simulink model "simulation_PID"  (R2020a)
settings: Solver=VariableStepAuto  StartTime=0.0  StopTime=100  RelTol=1e-3
libraries: simulink x1
settings Model: Creator=Ayush Agrawal  LastModifiedBy=Ayush Agrawal

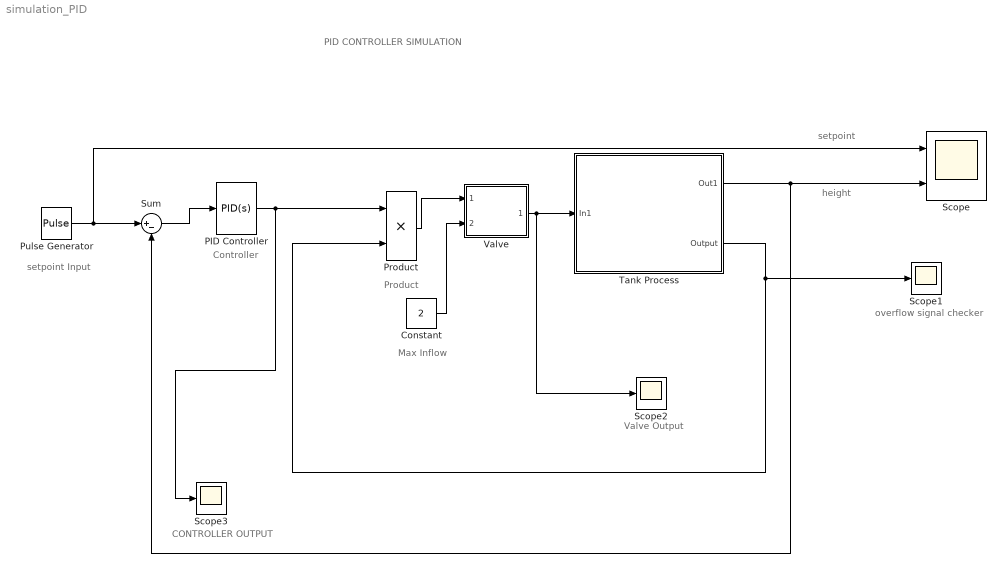
== system simulation_PID ==
  note: PID CONTROLLER SIMULATION
  note: CONTROLLER OUTPUT
  note: Product
  note: Controller
  note: Valve Output
  note: setpoint Input
  note: Max Inflow
  note: height
  note: setpoint
  note: overflow signal checker
  Constant : Constant  Value=2
  PID Controller : simulink/Continuous/PID Controller  Controller=PID  Form=Parallel  TimeDomain=Continuous-time  UseExternalTs=off  SampleTime=-1  IntegratorMethod=Forward Euler  FilterMethod=Forward Euler  ControllerParametersSource=internal  P=160  I=-2.93  D=16  UseFilter=on  N=100  TunerSelectOption=Transfer Function Based (PID Tuner App)  InitialConditionSource=internal  InitialConditionForIntegrator=0  InitialConditionForFilter=0  DifferentiatorICPrevScaledInput=0  ExternalReset=none  TrackingMode=off  Kt=1  LimitOutput=off  UpperSaturationLimit=inf  LowerSaturationLimit=-inf  LinearizeAsGain=on  AntiWindupMode=none  Kb=1  POutMin=[]  POutMax=[]  IOutMin=[]  IOutMax=[]  DOutMin=[]  DOutMax=[]  NOutMin=[]  NOutMax=[]  SumOutMin=[]  SumOutMax=[]  SaturationOutMin=[]  SaturationOutMax=[]  PParamMin=[]  PParamMax=[]  IParamMin=[]  IParamMax=[]  DParamMin=[]  DParamMax=[]  NParamMin=[]  NParamMax=[]  KbParamMin=[]  KbParamMax=[]  KtParamMin=[]  KtParamMax=[]  KbOutMin=[]  KbOutMax=[]  KtOutMin=[]  KtOutMax=[]  IntegratorOutMin=[]  IntegratorOutMax=[]  FilterOutMin=[]  FilterOutMax=[]  SumI1OutMin=[]  SumI1OutMax=[]  SumI2OutMin=[]  SumI2OutMax=[]  SumI3OutMin=[]  SumI3OutMax=[]  SumI4OutMin=[]  SumI4OutMax=[]  SumDOutMin=[]  SumDOutMax=[]  DifferentiatorOutMin=[]  DifferentiatorOutMax=[]  FilterDiffOutCoefMin=[]  FilterDiffOutCoefMax=[]  ReciprocalOutMin=[]  ReciprocalOutMax=[]  SumDenOutMin=[]  SumDenOutMax=[]  SumNumOutMin=[]  SumNumOutMax=[]  DivideOutMin=[]  DivideOutMax=[]  UdiffTsProdOutMin=[]  UdiffTsProdOutMax=[]  NTsProdOutMin=[]  NTsProdOutMax=[]  UintegralTsProdOutMin=[]  UintegralTsProdOutMax=[]  UngainTsProdOutMin=[]  UngainTsProdOutMax=[]  IntegratorContinuousStateAttributes=''  IntegratorStateMustResolveToSignalObject=off  IntegratorRTWStateStorageClass=Auto  FilterContinuousStateAttributes=''  FilterStateMustResolveToSignalObject=off  FilterRTWStateStorageClass=Auto  ParallelPVariant=InternalParameters  IdealPVariant=Disabled  IVariant=InternalParameters  DVariant=InternalParameters  IntegratorVariant=Continuous  SatVariant=Disabled  AWVariant=Passthrough  PCopyVariant=Disabled  TRVariant=Disabled  FdbkBlocksVariant=Forward  IdealPFdbkVariant=Disabled  SatFdbkVariant=Disabled  DerivativeFilterVariant=ContFilter  NVariant=InternalParameters  NCopyVariant=Disabled  FilterICVariant=InternalICsFilter  IntegratorICVariant=InternalICs  ExternalResetVariant=Disabled  TRSumVariant=Passthrough  SumFdbkVariant=Disabled  SumVariant=Sum_PID  TsampFilterVariant=InternalTs  TsampNgainVariant=Passthrough  TsampIntegralVariant=Passthrough
  Product : Product
  Pulse Generator : DiscretePulseGenerator  PulseType=Time based  Period=100  PulseWidth=50
  Scope : Scope  NumInputPorts=2
  Scope1 : Scope
  Scope2 : Scope
  Scope3 : Scope
  Sum : Sum  Inputs=|+-
  Tank Process : Subsystem  mask{ht=10, Tarea=0.4, Oarea=0.04, initialHt=0.0, overflowLimit=0}
      mask prompts: ht "Height of Tank(m)"; Tarea "Tank Area (m^2)"; Oarea "Outflow Cross-Section Area(m^2)"; initialHt "Initial Level Height(m)"; overflowLimit "Overflow Sensor distance from top(m)"
      mask Display: image('C:\Users\Ayush Agrawal\Downloads\94-943202_intermediate-practice-problems-online-brilliant-you-filling-water.png'); % Use "Edit Image" on toolstrip to change.
  Valve : Subsystem  mask(Valve){InitialPosition=0}
      mask prompts: InitialPosition "Initial position [0=closed 1=open]:"
      mask help: Valve
      mask Display: disp('VALVE')
  wires:
  Pulse Generator/1 -> Sum/1, Scope/1
  Tank Process/1(Out1) -> Sum/2, Scope/2
  Sum/1 -> PID Controller/1
  Tank Process/2(Output) -> Product/2, Scope1/1
  PID Controller/1 -> Scope3/1, Product/1
  Product/1 -> Valve/1(control)
  Valve/1(out flow) -> Scope2/1, Tank Process/1(In1)
  Constant/1 -> Valve/2(source flow)

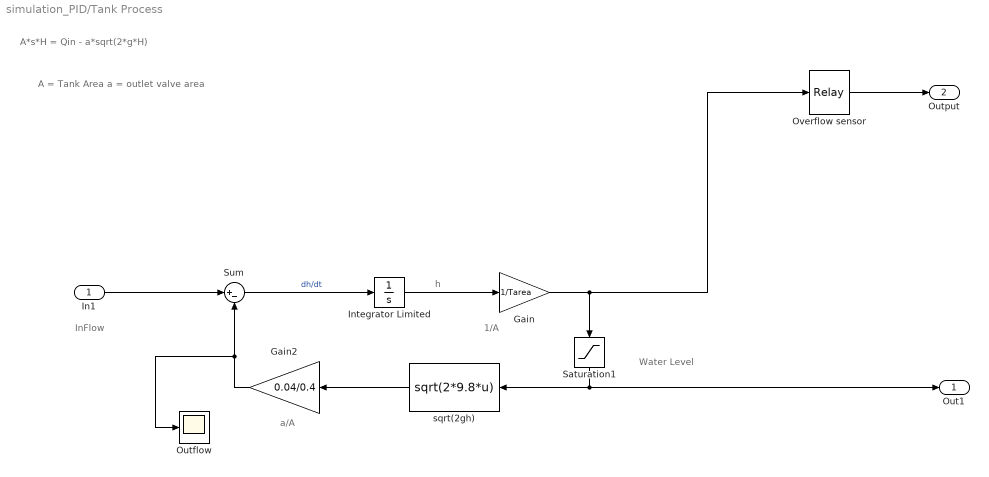
== system simulation_PID/Tank Process ==
  note: 1/A
  note: A = Tank Area
      | a = outlet valve area
  note: h
  note: A*s*H = Qin - a*sqrt(2*g*H)
  note: a/A
  note: InFlow
  note: Water Level
  In1 : Inport
  Gain : Gain  Gain=1/Tarea
  Gain2 : Gain  Gain=0.04/0.4
  Integrator Limited : Integrator  LimitOutput=on  UpperSaturationLimit=ht*Tarea  LowerSaturationLimit=0
  Outflow : Scope
  Overflow sensor : Relay  OnSwitchValue=ht - overflowLimit  OffSwitchValue=0  OnOutputValue=0  OffOutputValue=1
  Saturation1 : Saturate  UpperLimit=10  LowerLimit=0  OutMin=0  OutMax=10
  Sum : Sum  Inputs=|+-
  sqrt(2gh) : Fcn  Expr=sqrt(2*9.8*u)
  Out1 : Outport
  Output : Outport  Port=2
  wires:
  Overflow sensor/1 -> Output/1
  In1/1 -> Sum/1
  Gain2/1 -> Outflow/1, Sum/2
  Gain/1 -> Overflow sensor/1, Saturation1/1
  Sum/1 -> Integrator Limited/1  "dh/dt"
  Integrator Limited/1 -> Gain/1
  Saturation1/1 -> sqrt(2gh)/1, Out1/1
  sqrt(2gh)/1 -> Gain2/1

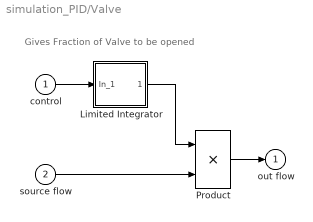
== system simulation_PID/Valve ==
  note: Gives Fraction of Valve to be opened
  control : Inport
  source flow : Inport  Port=2
  Limited Integrator : Subsystem  mask(Limited integrator.){lb=0, ub=1, xi=InitialPosition}
      mask prompts: lb "Lower bound:"; ub "Upper bound:"; xi "Initial condition"
      mask help: Limited integrator
      mask Help: Implements a limited integrator with \nan expression of the form:\n\nif(x<=lb and u<0) or (x>=ub and u>0)\n\txdot=0\nelse\n\txdot=u.
      mask Display: plot(-1,-0.2,3.5,1.2,[0.05,1,2,2.9],[0,0,1,1]);disp(' 1/s    ')
  Product : Product  InputSameDT=on  RndMeth=Zero  SaturateOnIntegerOverflow=on  OutDataTypeStr=Inherit: Same as first input
  out flow : Outport  InitialOutput=0  VectorParamsAs1DForOutWhenUnconnected=off
  wires:
  source flow/1 -> Product/2
  Product/1 -> out flow/1
  control/1 -> Limited Integrator/1(In_1)
  Limited Integrator/1(Out_1) -> Product/1

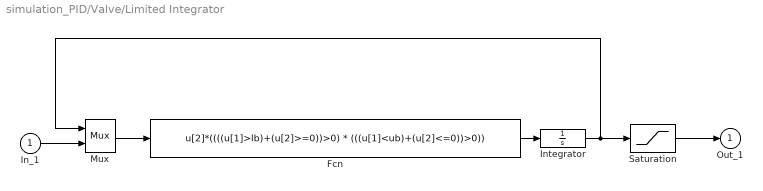
== system simulation_PID/Valve/Limited Integrator ==
  In_1 : Inport
  Fcn : Fcn  Expr=u[2]*((((u[1]>lb)+(u[2]>=0))>0) * (((u[1]<ub)+(u[2]<=0))>0))
  Integrator : Integrator  InitialCondition=xi
  Mux : Mux  Inputs=2
  Saturation : Saturate  UpperLimit=ub  LowerLimit=lb
  Out_1 : Outport  InitialOutput=0  VectorParamsAs1DForOutWhenUnconnected=off
  wires:
  Integrator/1 -> Saturation/1, Mux/1
  Fcn/1 -> Integrator/1
  Mux/1 -> Fcn/1
  In_1/1 -> Mux/2
  Saturation/1 -> Out_1/1
